simulink model "lr8"  (R2022a)
settings: Solver=VariableStepAuto  StartTime=0.0  StopTime=inf  RelTol=1e-3
InitFcn:
  | val = 149;
undefined symbols (not defined in the file): addr
libraries: instrumentseriallib x3
settings Model: Creator=User  LastModifiedBy=User

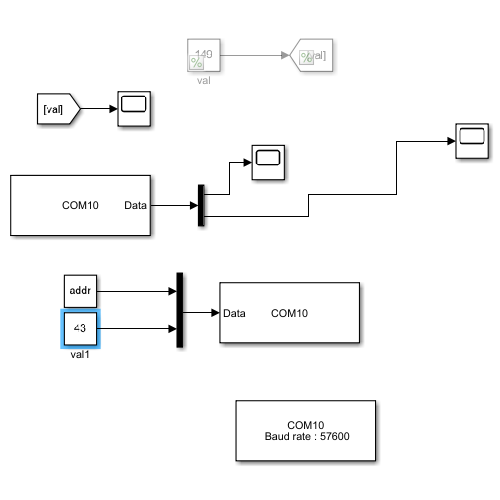
[thumbnail: Simulink's stored preview of the top-level diagram]
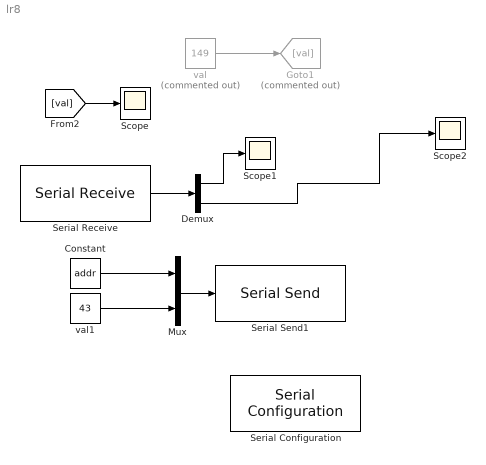
== system lr8 ==
  Constant : Constant  Value=addr
  Demux : Demux  Outputs=2
  Goto1 : Goto  Commented=on  GotoTag=val
  Mux : Mux  Inputs=2
  Scope : Scope
  Scope1 : Scope
  Scope2 : Scope
  Serial Configuration : instrumentseriallib/Serial Configuration  Priority=-200000  PortSel=COM10  Port=COM10  ComPort=COM10  BaudRate=57600  DataBits=8  Parity=none  StopBits=1  ByteOrder=little-endian  FlowControl=none  Timeout=1  SimulateUsing=Interpreted execution  BlockInModel=on  aMode=1
      settings: SourceProductBaseCode=OT,IC,MT
  Serial Receive : instrumentseriallib/Serial Receive  Priority=1  PortSel=COM10  Port=COM10  ComPort=COM10  DataType=uint16  SaveDataType=uint8  ToggleHeader=on  Header='rrrr'  ToggleTerminator=on  Terminator=Custom terminator  CustomTerminator='nnnn'  InputFormat=Row major  ToggleDataSize=on  DataSize=[2]  EnableBlockingMode=on  ActionDataUnavailable=Output custom value  ActionWhenDataUnavailable=Output custom value  CustomValue=-1  SampleTime=0.01  SimulateUsing=Interpreted execution  BlockInModel=on  aMode=1
      settings: SourceProductBaseCode=OT,IC,MT
  Serial Send1 : instrumentseriallib/Serial Send  Priority=1  PortSel=COM10  Port=COM10  ComPort=COM10  Header='rrrr'  Terminator=Custom terminator  CustomTerminator='nnnn'  EnableBlockingMode=on  SimulateUsing=Interpreted execution  BlockInModel=on  aMode=1
      settings: SourceProductBaseCode=OT,IC,MT
  val : Constant  Commented=on  Value=149  OutDataTypeStr=uint16  SampleTime=0.1
  val1 : Constant  Value=43  OutDataTypeStr=uint16  SampleTime=0.1
  wires:
  val/1 -> Goto1/1
  Mux/1 -> Serial Send1/1
  Serial Receive/1 -> Demux/1
  [val] -> Scope/1
  Demux/1 -> Scope1/1
  Demux/2 -> Scope2/1
  Constant/1 -> Mux/1
  val1/1 -> Mux/2
